simulink model "mat1_motor_drive_mega_V1_2019b"  (R2019b)
settings: Solver=FixedStepAuto  StartTime=0.0  StopTime=inf  RelTol=1e-3
libraries: arduinolib x4, simulink x1
settings Model: SILPILModeSetting=veronly  ExtModeTrigDuration=2  Creator=MU  LastModifiedBy=MU
settings DataIOCC: ReturnWorkspaceOutputs=off
settings OptimizationCC: DefaultUnderspecifiedDataType=single  EnhancedBackFolding=on  PassReuseOutputArgsAs=Individual arguments  ZeroExternalMemoryAtStartup=off  ZeroInternalMemoryAtStartup=off  MaxStackSize=64  OptimizeBlockOrder=speed  DifferentSizesBufferReuse=on  OptimizationCustomize=off  EfficientTunableParamExpr=on
settings DebuggingCC: ParameterTunabilityLossMsg=error
settings HardwareCC: ProdBitPerInt=16  ProdBitPerPointer=16  ProdBitPerSizeT=16  ProdBitPerPtrDiffT=16  ProdLargestAtomicFloat=None  ProdWordSize=8  ProdHWDeviceType=Atmel->AVR  UseEmbeddedCoderFeatures=off  UseSimulinkCoderFeatures=off
settings SFSimCC: MATLABDynamicMemAlloc=off
settings RTWCC: SystemTargetFile=ert.tlc  HardwareBoard=Arduino Mega 2560  TLCOptions=-aInlineSetEventsForThisBaseRateFcn=TLC_FALSE -aSuppressMultiTaskScheduler=TLC_FALSE -aRateBasedStepFcn=1  TemplateMakefile=ert_default_tmf  GenerateReport=on  Toolchain=Arduino AVR  BuildConfiguration=Faster Runs  IncludeHyperlinkInReport=on  LaunchReport=on  GenerateTraceInfo=on  GenerateTraceReport=on  GenerateTraceReportSl=on  GenerateTraceReportSf=on  GenerateTraceReportEml=on
settings CodeAppCC: ForceParamTrailComments=on  IgnoreCustomStorageClasses=off  OperatorAnnotations=on  SimulinkDataObjDesc=on  SFDataObjDesc=on  MangleLength=10  InsertBlockDesc=on
settings ERTTargetCC: SupportContinuousTime=on  SupportNonInlinedSFcns=on  SupportVariableSizeSignals=on  ExtModeStaticAllocSize=2048

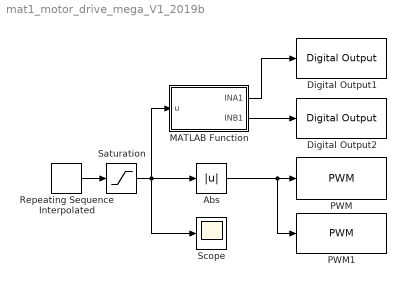
== system mat1_motor_drive_mega_V1_2019b ==
  Abs : Abs
  Digital Output1 : arduinolib/Digital Output  pinNumber=2  blockPlatform=arduino
  Digital Output2 : arduinolib/Digital Output  pinNumber=4  blockPlatform=arduino
  MATLAB Function : MATLAB Function  TreatAsAtomicUnit=on
  PWM : arduinolib/PWM  pinNumber=9  EnableInputFrequency=off  InitialFrequency=2000  InitialDutyCycle=0  NotificationType=None  blockPlatform=arduino
  PWM1 : arduinolib/PWM  pinNumber=13  EnableInputFrequency=off  InitialFrequency=2000  InitialDutyCycle=0  NotificationType=None  blockPlatform=arduino
  Repeating Sequence Interpolated : simulink/Sources/Repeating Sequence Interpolated  OutValues=[255 255 -255 -255 255 255 -255 -255 255 255 -255 -255 255 255 -255 -255].'  TimeValues=[0 1 1.001 2 2.001 3 3.001 4 4.001 5 5.001 6 6.001 7 7.001 8].'  LookUpMeth=Interpolation-Use End Values  tsamp=0.0025  OutMin=[]  OutMax=[]  OutDataTypeStr=double  OutputDataTypeScalingMode=double  OutDataType=fixdt(0,8)  OutScaling=2^-10
  Saturation : Saturate  UpperLimit=255  LowerLimit=-255
  Scope : Scope
  wires:
  Repeating Sequence Interpolated/1 -> Saturation/1
  MATLAB Function/1(INA1) -> Digital Output1/1
  Abs/1 -> PWM1/1, PWM/1
  MATLAB Function/2(INB1) -> Digital Output2/1
  Saturation/1 -> MATLAB Function/1(u), Scope/1, Abs/1

== matlab function mat1_motor_drive_mega_V1_2019b/MATLAB Function ==
  data: u input; INA1 output; INB1 output
function [INA1,INB1] = fcn(u)
 if(u<0) %CCW
    INA1 = 0;
    INB1 = 1;
 elseif(u==0) %STOP
    INA1 = 0;
    INB1 = 0;
 else %CW
    INA1 = 1;
    INB1 = 0;
 end
end
